simulink library "Ventilation_Window"  (Simulink 8.2)
settings: Solver=ode45  StartTime=0.0  StopTime=10.0  RelTol=1e-3
undefined symbols (not defined in the file): Ahabit, Hroom, rec, vent
libraries: carnot x2
settings Model: Creator=lena.frank  LastModifiedBy=drhf

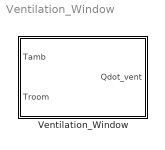
== system Ventilation_Window ==
  Ventilation_Window : Subsystem  mask(Ventilation with Heat Recovery and Window){vent=vent, rec=rec, Vhouse=Ahabit*Hroom}
      mask prompts: vent "Ventilation rate in 1/h"; rec "Heat recovery in 0..1"; Vhouse "Volume of the house"
      mask help:
      | Model of a mechanical ventilation system with heat recovery and a ventilation with windows.
      | The is suitable for the simple building model (see /Load/Houses/Simpe_House).
      mask init:
      | rec = max(0, min(1, rec));
      mask Help: web(fullfile(path_carnot('help'),'Ventilation_Window.html'),'-helpbrowser')
      mask Display: plot(0,10,90,80,[20 70 70 20 20],[20 20 70 70 20],[20 70 80 30 20],[20 20 65 65 20])

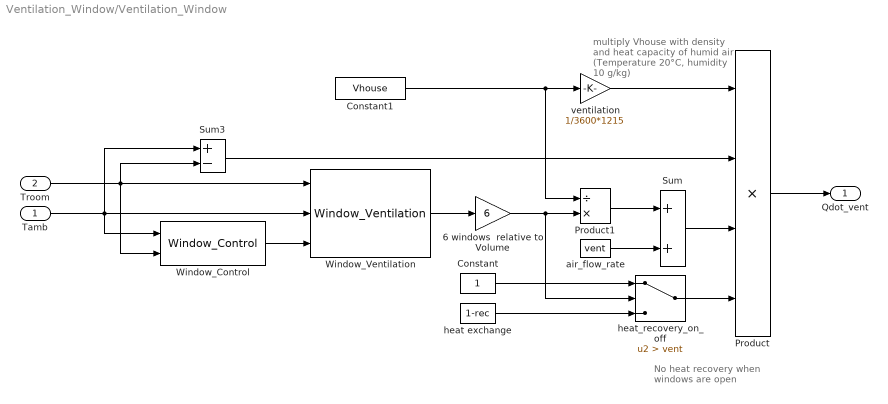
== system Ventilation_Window/Ventilation_Window ==
  note: No heat recovery
      | when windows are open
  note: multiply Vhouse with
      | density and heat capacity of humid air
      | (Temperature 20°C, humidity 10 g/kg)
  Tamb : Inport
  Troom : Inport  Port=2
  6 windows  relative to Volume : Gain  Gain=6
  Constant : Constant
  Constant1 : Constant  Value=Vhouse
  Product : Product  Inputs=4  RndMeth=Zero
  Product1 : Product  Inputs=/*  RndMeth=Zero
  Sum : Sum
  Sum3 : Sum  Inputs=+-  SaturateOnIntegerOverflow=on  InputSameDT=on  OutDataTypeStr=Inherit: Same as first input
  Window_Control : carnot/Control/Window_Control
  Window_Ventilation : carnot/Basic/Ventilation/Window_Ventilation  alpha=10  H=1  W=1
  air_flow_rate : Constant  Value=vent
  heat exchange : Constant  Value=1-rec
  heat_recovery_on_off : Switch  Criteria=u2 > Threshold  Threshold=vent
  ventilation : Gain  Gain=1/3600*1215  SaturateOnIntegerOverflow=on  OutDataTypeStr=Inherit: Same as input  ParamDataTypeStr=Inherit: Same as input
  Qdot_vent : Outport
  wires:
  heat_recovery_on_off/1 -> Product/4
  Constant/1 -> heat_recovery_on_off/1
  heat exchange/1 -> heat_recovery_on_off/3
  6 windows  relative to Volume/1 -> heat_recovery_on_off/2, Product1/2
  Sum/1 -> Product/3
  Product/1 -> Qdot_vent/1
  Constant1/1 -> Product1/1, ventilation/1
  ventilation/1 -> Product/1
  Sum3/1 -> Product/2
  Tamb/1 -> Window_Control/1, Window_Ventilation/2, Sum3/1
  Troom/1 -> Window_Control/2, Window_Ventilation/1, Sum3/2
  Product1/1 -> Sum/1
  air_flow_rate/1 -> Sum/2
  Window_Ventilation/1 -> 6 windows  relative to Volume/1
  Window_Control/1 -> Window_Ventilation/3
